simulink model "External_device"  (R2022b)
settings: Solver=ode1be  StartTime=0.0  StopTime=10.0  FixedStep=0.001  RelTol=1e-3
settings Model: Creator=Maxim Kozlov  LastModifiedBy=KozlovM
settings OptimizationCC: ReuseModelBlockBuffer=on

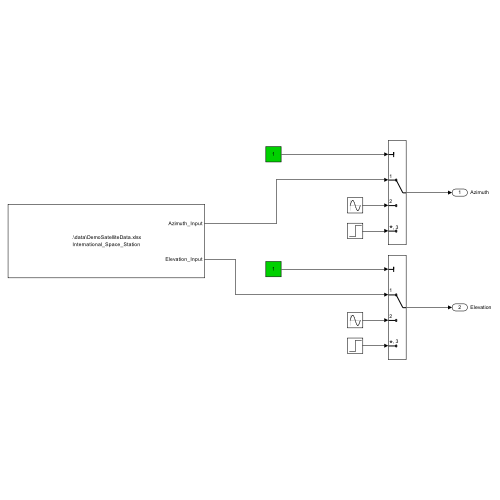
[thumbnail: Simulink's stored preview of the top-level diagram]
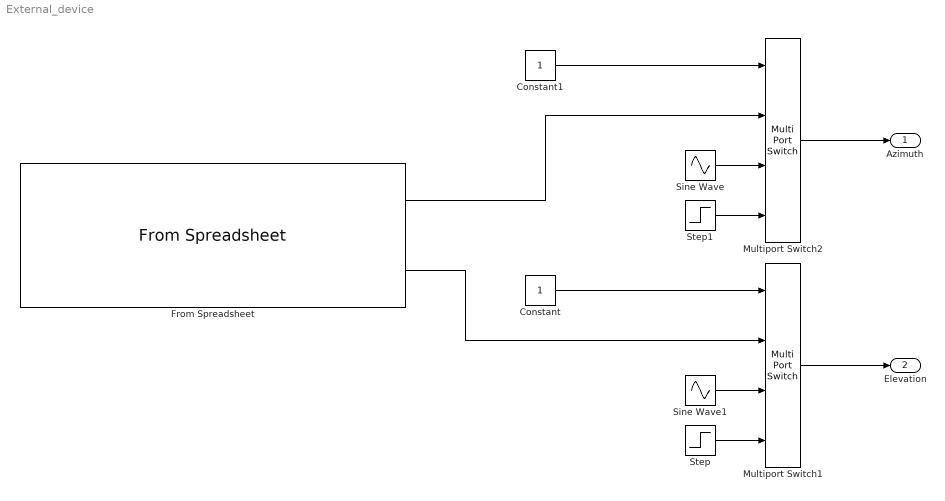
== system External_device ==
  Constant : Constant
  Constant1 : Constant
  From Spreadsheet : FromSpreadsheet  FileName=.\data\DemoSatelliteData.xlsx  SheetName=International_Space_Station
  Multiport Switch1 : MultiPortSwitch  SaturateOnIntegerOverflow=off  InputSameDT=off
  Multiport Switch2 : MultiPortSwitch  SaturateOnIntegerOverflow=off  InputSameDT=off
  Sine Wave : Sin  Amplitude=6  Frequency=0.5  Phase=pi/2  SampleTime=0
  Sine Wave1 : Sin  Amplitude=6  SampleTime=0
  Step : Step  SampleTime=0
  Step1 : Step  SampleTime=0
  Azimuth : Outport
  Elevation : Outport  Port=2
  wires:
  From Spreadsheet/2 -> Multiport Switch1/2
  Constant1/1 -> Multiport Switch2/1
  Step1/1 -> Multiport Switch2/4
  Sine Wave/1 -> Multiport Switch2/3
  Multiport Switch1/1 -> Elevation/1
  From Spreadsheet/1 -> Multiport Switch2/2
  Step/1 -> Multiport Switch1/4
  Sine Wave1/1 -> Multiport Switch1/3
  Constant/1 -> Multiport Switch1/1
  Multiport Switch2/1 -> Azimuth/1
